simulink model "Auto_Headlight_Control_openended"  (R2025b)
settings: Solver=VariableStepAuto  StartTime=0.0  StopTime=10  RelTol=1e-3
libraries: simulink x1
settings Model: Creator=spoor  LastModifiedBy=spoor

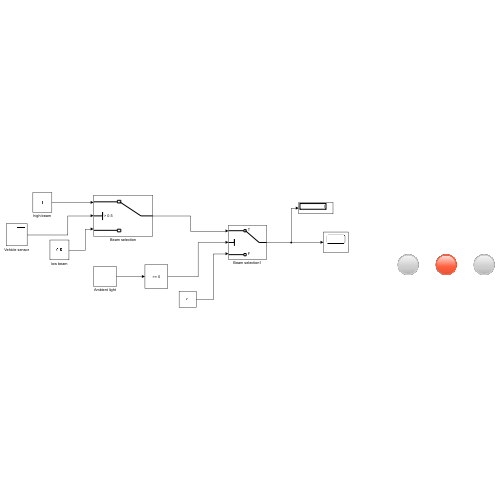
[thumbnail: Simulink's stored preview of the top-level diagram]
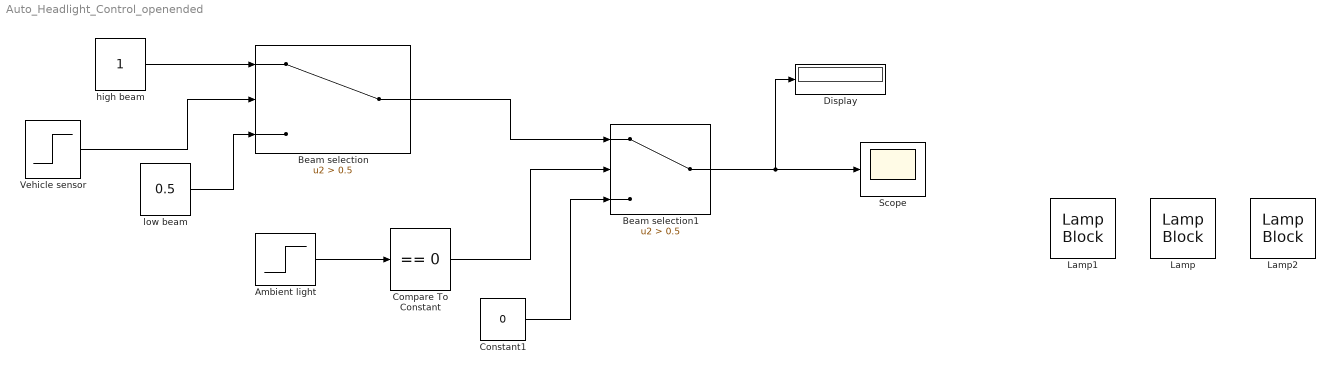
== system Auto_Headlight_Control_openended ==
  Ambient light : Step  Time=5  Before=1  After=0  SampleTime=0
  Beam selection : Switch  Criteria=u2 > Threshold  Threshold=0.5  SaturateOnIntegerOverflow=off  InputSameDT=off
  Beam selection1 : Switch  Criteria=u2 > Threshold  Threshold=0.5  SaturateOnIntegerOverflow=off  InputSameDT=off
  Compare To Constant : simulink/Logic and Bit Operations/Compare To Constant  relop===  const=0  OutDataTypeStr=boolean
  Constant1 : Constant  Value=0
  Display : Display
  Lamp : LampBlock  LabelPosition=Hide  DefaultColor=[192.0, 192.0, 192.0]
  Lamp1 : LampBlock  LabelPosition=Hide  DefaultColor=[192.0, 192.0, 192.0]
  Lamp2 : LampBlock  LabelPosition=Hide  DefaultColor=[192.0, 192.0, 192.0]
  Scope : Scope
      settings: ActiveDisplayYMinimum=-1  ActiveDisplayYMaximum=1
  Vehicle sensor : Step  Time=10  SampleTime=0
  high beam : Constant
  low beam : Constant  Value=0.5
  wires:
  high beam/1 -> Beam selection/1
  Vehicle sensor/1 -> Beam selection/2
  low beam/1 -> Beam selection/3
  Beam selection/1 -> Beam selection1/1
  Ambient light/1 -> Compare To Constant/1
  Compare To Constant/1 -> Beam selection1/2
  Constant1/1 -> Beam selection1/3
  Beam selection1/1 -> Display/1, Scope/1
